simulink model "NXT_test"  (Simulink 7.6)
settings: Solver=FixedStepDiscrete  StartTime=0.0  StopTime=Inf  RelTol=1e-3
libraries: rpi_blkst x1
settings Model: Creator=jacques  LastModifiedBy=jacques  SimulationMode=external
settings OptimizationCC: OptimizeModelRefInitCode=on  LifeSpan=1
settings HardwareCC: ProdIntDivRoundTo=Zero  ProdEndianess=LittleEndian  ProdHWDeviceType=Intel->x86/Pentium
settings RTWCC: SystemTargetFile=ert_rpi.tlc  TemplateMakefile=ert_rpi.tmf  PostCodeGenCommand=postGenFunc(buildInfo)  Description=RTW Embedded Coder RPI target  ProcessScript=ert_rpi_make_rtw_hook
settings CodeAppCC: IgnoreCustomStorageClasses=off
settings STFCustomTargetCC: ModelReferenceCompliant=off  CombineOutputUpdateFcns=on  ERTCustomFileBanners=on  SupportNonInlinedSFcns=off  SystemTargetFile=ert_rpi.tlc
settings ERTTargetCC: MultiwordLength=2048  ModelReferenceCompliant=off  ParMdlRefBuildCompliant=off  CompOptLevelCompliant=off  ERTFirstTimeCompliant=off  SupportContinuousTime=on  ModelStepFunctionPrototypeControlCompliant=off  CPPClassGenCompliant=off  ExtMode=on  ExtModeMexArgs='192.168.2.1'  InlinedParameterPlacement=NonHierarchical  ERTCustomFileTemplate=ert_rpi_file_process.tlc  ConvertIfToSwitch=off

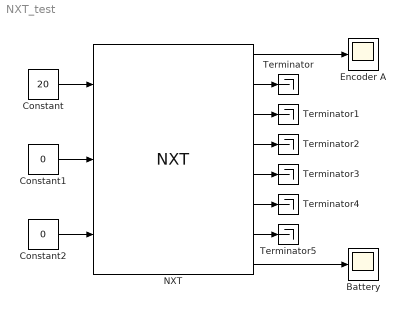
== system NXT_test ==
  Battery : Scope
      settings: YMin=8610  YMax=8700
  Constant : Constant  Value=20  SampleTime=0.01
  Constant1 : Constant  Value=0  SampleTime=0.01
  Constant2 : Constant  Value=0  SampleTime=0.01
  Encoder A : Scope
      settings: YMin=1800  YMax=2900
  NXT : rpi_blkst/NXT  SystemSampleTime=-1  rpi_mask_Ts=0.01  rpi_mask_id=1
  Terminator{,1..5} (6 alike) : Terminator
  wires:
  Constant/1 -> NXT/1
  Constant1/1 -> NXT/2
  Constant2/1 -> NXT/3
  NXT/2 -> Terminator/1
  NXT/3 -> Terminator1/1
  NXT/4 -> Terminator2/1
  NXT/5 -> Terminator3/1
  NXT/6 -> Terminator4/1
  NXT/7 -> Terminator5/1
  NXT/1 -> Encoder A/1
  NXT/8 -> Battery/1
